simulink model "PubIfDecisionLM_MDL"  (R2020b)
settings: configuration reference "DspaceConfig" (kept outside this file)
PostLoadFcn:
  | if any(exist('dsrtsu_mdlpostloadfcn', 'file') ~= 0), dsrtsu_mdlpostloadfcn('Execute', bdroot); end
InitFcn:
  | , if any(exist('dsmpb_private', 'file') ~= 0), dsmpb_private('dsmpb_mdlclblib', 'Init', bdroot); end,
undefined symbols (not defined in the file or in its folder): OFM_OBJ_FUSIONTYPE_E, OFM_OBJ_MOVINGSTATE_E, OFM_OBJ_ORIENTATION_E, OFM_OBJ_TYPE_E, P_LM_Cyc, P_LM_EMLHistKapRcdBufSize, P_LM_EMLHistTrajBaseDis, P_LM_EMLHistTrajPNum, P_LM_EMLKapCorrMaxThre, P_LM_EMLMinKapThre, P_LM_EMLPathDisDiffThre, P_LM_EMLQuaFiltPar, P_LM_EMLTurnActKapThre, P_LM_EMLValidQuaThre, P_LM_FntPath1Disgap, P_LM_FntPath1MinDis, P_LM_FntPath1Timegap, P_LM_FntPath2Disgap, P_LM_FntPath2MinDis, P_LM_FntPath2Timegap, P_LM_FntPath3Disgap, P_LM_FntPath3MinDis, P_LM_FntPath3Timegap, P_LM_FusBLParFiltP, P_LM_FusEVDifC2Thre, P_LM_FusEVOPath1AllVSLDisThre, P_LM_FusEVOPath1AllVSLLostNumThre, P_LM_FusEVOPath1AllVSLQuaThre, P_LM_FusEVOPath1OTLFacNLC, P_LM_FusOTLQuaThre, P_LM_FusOTLSW, P_LM_FusParC0Index, P_LM_FusParC1Index, P_LM_FusParC2Index, P_LM_FusParC3Index, P_LM_FusVSLQuaThre, P_LM_FusVSLSW, P_LM_FusVSLValidSteerWheerAngThre, P_LM_FusVSLValidVxvThre, P_LM_LaneWidth, P_LM_OTLBufTPInfoEvaFactor, P_LM_OTLObjNum, P_LM_OTLObjSelectAgeThre, P_LM_OTLObjSelectDxAssessVx, P_LM_OTLObjSelectDxThre, P_LM_OTLObjSelectVxThre, P_LM_OTLObjSelectVyAssessDx, P_LM_OTLObjSelectVyThre, P_LM_OTLTrajPntBaseDis, P_LM_OTLTrajStdThre, P_LM_VSLAvailLineNum, P_LM_VSLBLSDiffThre, P_LM_VSLBLSDisRatio, P_LM_VSLFusBLParFiltP_C1, P_LM_VSLFusBLParFiltP_C2, P_LM_VSLFusBLParFiltP_C3, P_LM_VSLFusBLParFiltP_Quality, P_LM_VSLHistTrajBaseDis, P_LM_VSLHistTrajPNum, P_LM_VSLLCC0diff ... (+18)
libraries: simulink x145, LM_LIB x43
(part 10 of 24)

== system PubIfDecisionLM_MDL/Subsystem2/LM_SigPrePro1/Subsystem1/Subsystem/Subsystem2 ==
  RFM_LINE : Inport
  Bus Creator : BusCreator  Inputs=13
  Bus Selector : BusSelector  OutputSignals=dC0V
  Bus Selector1 : BusSelector  OutputSignals=bIsLineExist,dC1V,dC2V,dC3V,dLaneWidth,eLineType,dDisStart,dDisFront,dQuality,eColour,eFuType,nTrackAge
  Constant4 : Constant  Value=P_LM_VSLMinLINEL2  OutDataTypeStr=single
  Constant5 : Constant  Value=P_LM_VSLMaxLINEL2  OutDataTypeStr=single
  Constant8 : Constant  Value=0  OutDataTypeStr=single
  Logical Operator : Logic  AllPortsSameDT=off  OutDataTypeStr=boolean
  Relational Operator : RelationalOperator  OutDataTypeStr=boolean  RndMeth=Simplest
  Relational Operator1 : RelationalOperator  Operator=<=  OutDataTypeStr=boolean  RndMeth=Simplest
  Switch : Switch  Criteria=u2 > Threshold
  RFM_LINE_L2 : Outport
  wires:
  Relational Operator1/1 -> Logical Operator/2
  Bus Selector1/6 -> Bus Creator/7  "<eLineType>"
  Bus Selector1/8 -> Bus Creator/9  "<dDisFront>"
  Bus Selector1/5 -> Bus Creator/6  "<dLaneWidth>"
  Bus Selector1/9 -> Bus Creator/10  "<dQuality>"
  RFM_LINE/1 -> Bus Selector/1, Bus Selector1/1
  Logical Operator/1 -> Switch/2
  Bus Selector1/1 -> Bus Creator/1  "<bIsLineExist>"
  Bus Selector1/10 -> Bus Creator/11  "<eColour>"
  Bus Selector1/7 -> Bus Creator/8  "<dDisStart>"
  Bus Selector/1 -> Relational Operator1/1, Relational Operator/1, Switch/1  "<dC0V>"
  Switch/1 -> [dC0V]  "dC0V"
  Bus Selector1/3 -> Bus Creator/4  "<dC2V>"
  Bus Selector1/4 -> Bus Creator/5  "<dC3V>"
  Constant5/1 -> Relational Operator1/2
  Relational Operator/1 -> Logical Operator/1
  Constant8/1 -> Switch/3
  Bus Selector1/2 -> Bus Creator/3  "<dC1V>"
  [dC0V] -> Bus Creator/2  "dC0V"
  Constant4/1 -> Relational Operator/2
  Bus Creator/1 -> RFM_LINE_L2/1
  Bus Selector1/11 -> Bus Creator/12  "<eFuType>"
  Bus Selector1/12 -> Bus Creator/13  "<nTrackAge>"

== system PubIfDecisionLM_MDL/Subsystem2/LM_SigPrePro1/Subsystem1/Subsystem/Subsystem3 ==
  RFM_LINE : Inport
  Bus Creator : BusCreator  Inputs=13
  Bus Selector : BusSelector  OutputSignals=dC0V
  Bus Selector1 : BusSelector  OutputSignals=bIsLineExist,dC1V,dC2V,dC3V,dLaneWidth,eLineType,dDisStart,dDisFront,dQuality,eColour,eFuType,nTrackAge
  Constant6 : Constant  Value=P_LM_VSLMinLINER2  OutDataTypeStr=single
  Constant7 : Constant  Value=P_LM_VSLMaxLINER2  OutDataTypeStr=single
  Constant8 : Constant  Value=0  OutDataTypeStr=single
  Logical Operator : Logic  AllPortsSameDT=off  OutDataTypeStr=boolean
  Relational Operator : RelationalOperator  OutDataTypeStr=boolean  RndMeth=Simplest
  Relational Operator1 : RelationalOperator  Operator=<=  OutDataTypeStr=boolean  RndMeth=Simplest
  Switch : Switch  Criteria=u2 > Threshold
  RFM_LINE_R2 : Outport
  wires:
  Bus Creator/1 -> RFM_LINE_R2/1
  Constant6/1 -> Relational Operator/2
  [dC0V] -> Bus Creator/2  "dC0V"
  Bus Selector1/2 -> Bus Creator/3  "<dC1V>"
  Constant8/1 -> Switch/3
  Relational Operator/1 -> Logical Operator/1
  Constant7/1 -> Relational Operator1/2
  Bus Selector1/4 -> Bus Creator/5  "<dC3V>"
  Bus Selector1/3 -> Bus Creator/4  "<dC2V>"
  Switch/1 -> [dC0V]  "dC0V"
  Bus Selector/1 -> Switch/1, Relational Operator/1, Relational Operator1/1  "<dC0V>"
  Bus Selector1/7 -> Bus Creator/8  "<dDisStart>"
  Bus Selector1/10 -> Bus Creator/11  "<eColour>"
  Bus Selector1/1 -> Bus Creator/1  "<bIsLineExist>"
  Logical Operator/1 -> Switch/2
  RFM_LINE/1 -> Bus Selector1/1, Bus Selector/1
  Bus Selector1/9 -> Bus Creator/10  "<dQuality>"
  Bus Selector1/5 -> Bus Creator/6  "<dLaneWidth>"
  Bus Selector1/8 -> Bus Creator/9  "<dDisFront>"
  Bus Selector1/6 -> Bus Creator/7  "<eLineType>"
  Relational Operator1/1 -> Logical Operator/2
  Bus Selector1/11 -> Bus Creator/12  "<eFuType>"
  Bus Selector1/12 -> Bus Creator/13  "<nTrackAge>"

== system PubIfDecisionLM_MDL/Subsystem2/LM_VSL/LM_VSLFntPath/LM_VSL_LineInfoEvalutaion/LM_VSL_BaseLinePCalc3 ==
  LM_ComLineLostNum : Inport
  LM_VSLLineQualityVect : Inport  Port=2
  LM_VSLLineC1Vect : Inport  Port=3
  LM_VSLLineC2Vect : Inport  Port=4
  LM_VSLLineC3Vect : Inport  Port=5
  LM_VSLLineMaxQualityIndex : Inport  Port=6
  LM_VSLLineMinQualityIndex : Inport  Port=7
  Diffnum : Inport  Port=8
  LM_VSLMinQualityLineValid : Inport  Port=9
  LM_VSLDiffValid : Inport  Port=10
  LM_VSLBLFntDis : Inport  Port=11
  LM_VSLLineDisFntVect : Inport  Port=12
  Subsystem : Subsystem
  Subsystem1 : Subsystem
  LM_VSLBaseC1 : Outport
  LM_VSLBaseC2 : Outport  Port=2
  LM_VSLBaseC3 : Outport  Port=3
  LM_VSLBaseQuality : Outport  Port=4
  wires:
  LM_VSLBLFntDis/1 -> Subsystem/12(LM_VSLBLFntDis)
  LM_VSLLineDisFntVect/1 -> Subsystem/11(LM_VSLLineDisFntVect)
  Subsystem1/4(LM_VSLBaseQualityFilt) -> LM_VSLBaseQuality/1  "LM_VSLBaseQualityFilt"
  Subsystem1/3(LM_VSLBaseC3Filt) -> LM_VSLBaseC3/1  "LM_VSLBaseC3Filt"
  Subsystem1/2(LM_VSLBaseC2Filt) -> LM_VSLBaseC2/1  "LM_VSLBaseC2Filt"
  Subsystem1/1(LM_VSLBaseC1Filt) -> LM_VSLBaseC1/1  "LM_VSLBaseC1Filt"
  Subsystem/4(LM_VSLBaseQuality) -> Subsystem1/4(LM_VSLBaseQuality)  "LM_VSLBaseQuality"
  Subsystem/3(LM_VSLBaseC3) -> Subsystem1/3(LM_VSLBaseC3)  "LM_VSLBaseC3"
  Subsystem/2(LM_VSLBaseC2) -> Subsystem1/2(LM_VSLBaseC2)  "LM_VSLBaseC2"
  Subsystem/1(LM_VSLBaseC1) -> Subsystem1/1(LM_VSLBaseC1)  "LM_VSLBaseC1"
  LM_VSLLineMaxQualityIndex/1 -> Subsystem/1(LM_VSLLineMaxQualityIndex)
  LM_VSLLineQualityVect/1 -> Subsystem/7(LM_VSLLineQualityVect)
  LM_VSLMinQualityLineValid/1 -> Subsystem/10(LM_VSLMinQualityLineValid)
  LM_VSLLineC1Vect/1 -> Subsystem/4(LM_VSLLineC1Vect)
  LM_VSLLineC2Vect/1 -> Subsystem/5(LM_VSLLineC2Vect)
  LM_VSLLineC3Vect/1 -> Subsystem/6(LM_VSLLineC3Vect)
  LM_ComLineLostNum/1 -> Subsystem/3(LM_ComLineLostNum)
  LM_VSLLineMinQualityIndex/1 -> Subsystem/2(LM_VSLLineMinQualityIndex)
  LM_VSLDiffValid/1 -> Subsystem/9(LM_VSLDiffValid)
  Diffnum/1 -> Subsystem/8(Diffnum)

== system PubIfDecisionLM_MDL/Subsystem2/LM_VSL/LM_VSLFntPath/LM_VSL_LineInfoEvalutaion/LM_VSL_LineInfoEvalutaion ==
  LM_ComLineLostNum : Inport
  LM_VSLLineQualityVect : Inport  Port=2
  LM_VSLLineC1Vect : Inport  Port=3
  LM_VSLLineC2Vect : Inport  Port=4
  LM_VSLLineC3Vect : Inport  Port=5
  LM_VSLLineC0Vect : Inport  Port=6
  LM_ComAllLineLost_flg : Inport  Port=7
  LM_VSLLineExistVect : Inport  Port=8
  LM_VSLLineDisFntVect : Inport  Port=9
  LM_VSL_LineDiffEvalutaion : Subsystem
  LM_VSL_LineDisEvaluation : Subsystem
  LM_VSL_LineQualityEvalutaion : Subsystem
  LM_VSLLineMaxQualityIndex : Outport
  LM_VSLLineMinQualityIndex : Outport  Port=2
  Diffnum : Outport  Port=3
  LM_VSLMinQualityLineValid : Outport  Port=4
  LM_VSLDiffValid : Outport  Port=5
  LM_VSLBLFntDis : Outport  Port=6
  LM_VSLLineMaxDis : Outport  Port=7
  wires:
  LM_VSL_LineDiffEvalutaion/3(LM_VSLBLFntDis) -> LM_VSLBLFntDis/1
  LM_VSL_LineDisEvaluation/1(LM_VSLLineMaxDis) -> [LM_VSLLineMaxDis], LM_VSLLineMaxDis/1
  LM_ComAllLineLost_flg/1 -> LM_VSL_LineDisEvaluation/1(LM_ComAllLineLost_flg), LM_VSL_LineQualityEvalutaion/1(LM_ComAllLineLost_flg)
  LM_VSLLineQualityVect/1 -> LM_VSL_LineQualityEvalutaion/3(LM_VSLLineQualityVect), LM_VSL_LineDiffEvalutaion/2(LM_VSLLineQualityVect)
  LM_VSL_LineQualityEvalutaion/2(LM_VSLLineMaxQualityIndex) -> [LM_VSLLineMaxQualityIndex], LM_VSLLineMaxQualityIndex/1
  LM_VSL_LineQualityEvalutaion/1(LM_VSLLineMinQualityIndex) -> LM_VSLLineMinQualityIndex/1
  LM_ComLineLostNum/1 -> LM_VSL_LineDiffEvalutaion/4(LM_ComLineLostNum)
  LM_VSLLineC1Vect/1 -> LM_VSL_LineDiffEvalutaion/6(LM_VSLLineC1Vect)
  LM_VSLLineC2Vect/1 -> LM_VSL_LineDiffEvalutaion/7(LM_VSLLineC2Vect)
  LM_VSLLineC3Vect/1 -> LM_VSL_LineDiffEvalutaion/8(LM_VSLLineC3Vect)
  LM_VSL_LineDiffEvalutaion/1("Diffnum ") -> Diffnum/1
  LM_VSL_LineDiffEvalutaion/2(LM_VSLDiffValid) -> LM_VSLDiffValid/1
  LM_VSLLineC0Vect/1 -> LM_VSL_LineDiffEvalutaion/5(LM_VSLLineC0Vect)
  LM_VSLLineExistVect/1 -> LM_VSL_LineDisEvaluation/2(LM_VSLLineExistVect), LM_VSL_LineDiffEvalutaion/1(LM_VSLLineExistVect), LM_VSL_LineQualityEvalutaion/2(LM_VSLLineExistVect)
  LM_VSLLineDisFntVect/1 -> LM_VSL_LineDisEvaluation/3(LM_VSLLineDisFntVect), LM_VSL_LineDiffEvalutaion/3(LM_VSLLineDisFntVect)
  LM_VSL_LineQualityEvalutaion/3(LM_VSLLineMaxQuality) -> [LM_VSLLineMaxQuality]
  LM_VSL_LineDisEvaluation/2(LM_VSLLineMaxDisIndex) -> [LM_VSLLineMaxDisIndex]
  [LM_VSLLineMaxDisIndex] -> LM_VSL_LineDiffEvalutaion/11(LM_VSLLineMaxDisIndex)
  [LM_VSLLineMaxDis] -> LM_VSL_LineDiffEvalutaion/10(LM_VSLLineMaxDis)
  [LM_VSLLineMaxQualityIndex] -> LM_VSL_LineDiffEvalutaion/12(LM_VSLLineMaxQualityIndex)
  [LM_VSLLineMaxQuality] -> LM_VSL_LineDiffEvalutaion/9(LM_VSLLineMaxQuality)
  LM_VSL_LineQualityEvalutaion/4(LM_VSLMinQualityLineValid) -> LM_VSLMinQualityLineValid/1

== system PubIfDecisionLM_MDL/Subsystem2/LM_VSL/LM_VSLFntPath/LM_VSL_LineQualityCalc/LM_VSL_FntPath1QualityCalc ==
  LM_VSLBaseDisAdju : Inport
  LM_FntPath1Dis : Inport  Port=2
  LM_VSLBaseQuality : Inport  Port=3
  Divide : Product  Inputs=*/
  Product : Product
  Saturation : Saturate  UpperLimit=1  LowerLimit=0
  Saturation1 : Saturate  UpperLimit=1  LowerLimit=0
  Saturation2 : Saturate  UpperLimit=70  LowerLimit=5
  LM_VSLFntPath1Quality : Outport
  wires:
  Saturation2/1 -> Divide/1
  LM_FntPath1Dis/1 -> Divide/2
  Product/1 -> Saturation/1
  LM_VSLBaseDisAdju/1 -> Saturation2/1
  Saturation/1 -> LM_VSLFntPath1Quality/1  "LM_VSLFntPath1Quality"
  Saturation1/1 -> Product/1
  LM_VSLBaseQuality/1 -> Product/2
  Divide/1 -> Saturation1/1

== system PubIfDecisionLM_MDL/Subsystem2/LM_VSL/LM_VSLFntPath/LM_VSL_LineQualityCalc/LM_VSL_FntPath2QualityCalc ==
  LM_FntPath1Dis : Inport
  LM_VSLBaseQuality : Inport  Port=2
  LM_VSLBaseDis : Inport  Port=3
  LM_FntPath2Dis : Inport  Port=4
  Chart : Stateflow chart  TreatAsAtomicUnit=on
  Constant2 : Constant  Value=P_LM_VSLPath1DisDiffThre
  Signal Conversion : SignalConversion  OverrideOpt=off
  LM_VSLFntPath2Quality : Outport
  wires:
  Signal Conversion/1 -> LM_VSLFntPath2Quality/1  "LM_VSLFntPath2Quality"
  LM_FntPath2Dis/1 -> Chart/2(LM_FntPath2Dis)
  LM_VSLBaseQuality/1 -> Chart/4(LM_VSLBaseQuality)
  LM_VSLBaseDis/1 -> Chart/1(LM_VSLBaseDis)
  LM_FntPath1Dis/1 -> Chart/3(LM_FntPath1Dis)
  Constant2/1 -> Chart/5(P_LM_PathDisDiffThre)
  Chart/1(pathquality) -> Signal Conversion/1

== system PubIfDecisionLM_MDL/Subsystem2/LM_VSL/LM_VSLFntPath/LM_VSL_LineQualityCalc/LM_VSL_FntPath2QualityCalc1 ==
  note: 为了防止第二段轨迹短暂丢失，该处设计逻辑为当上一周期存在第二段，但本周期车道线长度不足输出第二段，会对第二段延迟半秒时间
  note: 为了避免车道线最大长度跳变导致一会儿有第2段一会儿又没第2段，可能会导致目标跳变，该处加入有效性校验，即第2段延后0.5s放出
  LM_FntPath1Dis : Inport
  LM_VSLBaseQuality : Inport  Port=2
  LM_VSLBaseDis : Inport  Port=3
  LM_FntPath2Dis : Inport  Port=4
  Add : Sum
  Add1 : Sum
  Compare To Constant : simulink/Logic and Bit Operations/Compare To Constant  relop===  const=1  OutDataTypeStr=boolean
  Compare To Zero : simulink/Logic and Bit Operations/Compare To Zero  relop=~=  OutDataTypeStr=boolean
  Compare To Zero1 : simulink/Logic and Bit Operations/Compare To Zero  relop=~=  OutDataTypeStr=boolean
  Compare To Zero2 : simulink/Logic and Bit Operations/Compare To Zero  relop===  OutDataTypeStr=boolean
  Constant : Constant  Value=0  OutDataTypeStr=single
  Constant1 : Constant  OutDataTypeStr=uint8
  Constant2 : Constant  Value=-5
  Constant3 : Constant  Value=15  OutDataTypeStr=uint8
  Constant4 : Constant  Value=0  OutDataTypeStr=uint8
  Constant5 : Constant  Commented=on  Value=P_LM_EMLPathDisDiffThre
  Constant6 : Constant  OutDataTypeStr=uint8
  Constant7 : Constant  Value=25  OutDataTypeStr=uint8
  Constant8 : Constant  OutDataTypeStr=uint8
  Constant9 : Constant  Value=25  OutDataTypeStr=uint8
  Divide : Product  Inputs=*/
  Logical Operator : Logic  AllPortsSameDT=off  OutDataTypeStr=boolean
  Logical Operator1 : Logic  AllPortsSameDT=off  OutDataTypeStr=boolean
  Logical Operator2 : Logic  Operator=OR  AllPortsSameDT=off  OutDataTypeStr=boolean
  Logical Operator3 : Logic  AllPortsSameDT=off  OutDataTypeStr=boolean
  Product : Product
  Relational Operator : RelationalOperator  OutDataTypeStr=boolean  RndMeth=Nearest
  Relational Operator1 : RelationalOperator  OutDataTypeStr=boolean  RndMeth=Nearest
  Relational Operator2 : RelationalOperator  Operator=<  OutDataTypeStr=boolean  RndMeth=Nearest
  Saturation : Saturate  UpperLimit=1  LowerLimit=0
  Saturation1 : Saturate  UpperLimit=1  LowerLimit=0
  Saturation2 : Saturate  UpperLimit=255  LowerLimit=0
  Saturation3 : Saturate  UpperLimit=253  LowerLimit=0
  Scope6 : Scope
  Subtract : Sum  Inputs=+-
  Switch{3..7} (5 alike) : Switch  Criteria=u2 ~= 0
  Unit Delay : UnitDelay  SampleTime=-1  HasFrameUpgradeWarning=on
  Unit Delay1 : UnitDelay  SampleTime=-1  HasFrameUpgradeWarning=on
  Unit Delay2 : UnitDelay  SampleTime=-1  HasFrameUpgradeWarning=on
  LM_VSLFntPath2Quality : Outport
  wires:
  Product/1 -> Saturation/1
  Switch5/1 -> Saturation2/1, Unit Delay/1
  Unit Delay2/1 -> Add1/2
  LM_VSLBaseDis/1 -> Compare To Zero/1, Subtract/1, Divide/1
  Switch6/1 -> Compare To Constant/1
  Divide/1 -> Saturation1/1
  Switch3/1 -> LM_VSLFntPath2Quality/1  "LM_VSLFntPath2Quality"
  LM_VSLBaseQuality/1 -> Product/2
  Subtract/1 -> Relational Operator/1
  Constant3/1 -> Relational Operator1/2
  Constant/1 -> Switch3/3
  LM_FntPath1Dis/1 -> Subtract/2
  Switch4/1 -> Switch5/1
  Constant2/1 -> Relational Operator/2
  Saturation2/1 -> Relational Operator1/1
  Constant4/1 -> Switch5/3
  Add/1 -> Switch4/1
  Compare To Zero/1 -> Logical Operator/2
  Constant1/1 -> Add/1
  Saturation1/1 -> Product/1
  Logical Operator2/1 -> Switch3/2
  LM_FntPath2Dis/1 -> Divide/2
  Compare To Constant/1 -> Switch7/2
  Logical Operator3/1 -> Switch6/2
  Constant7/1 -> Switch6/3
  Unit Delay/1 -> Add/2, Switch4/3
  Constant6/1 -> Switch6/1
  Switch7/1 -> Saturation3/1
  Constant9/1 -> Relational Operator2/2
  Compare To Zero1/1 -> Logical Operator3/1
  Saturation3/1 -> Relational Operator2/1, Unit Delay2/1, Scope6/1
  Relational Operator2/1 -> Logical Operator2/1
  Logical Operator1/1 -> Unit Delay1/1, Compare To Zero2/1, Logical Operator2/2
  Compare To Zero2/1 -> Logical Operator3/2
  Constant8/1 -> Switch7/1, Add1/1
  Add1/1 -> Switch7/3
  Relational Operator/1 -> Logical Operator/1
  Unit Delay1/1 -> Compare To Zero1/1
  Saturation/1 -> Switch3/1  "LM_VSL_FntPath2_Quality"
  Relational Operator1/1 -> Logical Operator1/2
  Logical Operator/1 -> Switch4/2, Logical Operator1/1, Switch5/2

== system PubIfDecisionLM_MDL/Subsystem2/LM_VSL/LM_VSLFntPath/LM_VSL_LineQualityCalc/LM_VSL_FntPath3QualityCalc ==
  note: 为了避免车道线最大长度跳变导致一会儿有第三段一会儿又没第三段，可能会导致目标跳变，该处加入有效性校验，即第三段延后0.5s放出
  LM_FntPath2Dis : Inport
  LM_VSLBaseQuality : Inport  Port=2
  LM_VSLBaseDis : Inport  Port=3
  LM_FntPath3Dis : Inport  Port=4
  Chart : Stateflow chart  TreatAsAtomicUnit=on
  Constant1 : Constant  Value=P_LM_VSLPath2DisDiffThre
  Signal Conversion : SignalConversion  OverrideOpt=off
  LM_VSLFntPath3Quality : Outport
  wires:
  Signal Conversion/1 -> LM_VSLFntPath3Quality/1  "LM_VSLFntPath3Quality"
  Constant1/1 -> Chart/5(P_LM_PathDisDiffThre)
  LM_FntPath3Dis/1 -> Chart/3(LM_FntPath3Dis)
  LM_VSLBaseQuality/1 -> Chart/4(LM_VSLBaseQuality)
  LM_FntPath2Dis/1 -> Chart/2(LM_FntPath2Dis)
  LM_VSLBaseDis/1 -> Chart/1(LM_VSLBaseDis)
  Chart/1(pathquality) -> Signal Conversion/1

== system PubIfDecisionLM_MDL/Subsystem2/LM_VSL/LM_VSLFntPath/LM_VSL_LineQualityCalc/LM_VSL_FntPath3QualityCalc1 ==
  note: 为了防止第二段轨迹短暂丢失，该处设计逻辑为当上一周期存在第二段，但本周期车道线长度不足输出第二段，会对第二段延迟半秒时间
  note: 为了避免车道线最大长度跳变导致一会儿有第三段一会儿又没第三段，可能会导致目标跳变，该处加入有效性校验，即第三段延后0.5s放出
  LM_FntPath2Dis : Inport
  LM_VSLBaseQuality : Inport  Port=2
  LM_VSLBaseDis : Inport  Port=3
  LM_FntPath3Dis : Inport  Port=4
  Add : Sum
  Add1 : Sum
  Chart : Stateflow chart  TreatAsAtomicUnit=on
  Compare To Constant : simulink/Logic and Bit Operations/Compare To Constant  relop===  const=1  OutDataTypeStr=boolean
  Compare To Zero : simulink/Logic and Bit Operations/Compare To Zero  relop=~=  OutDataTypeStr=boolean
  Compare To Zero1 : simulink/Logic and Bit Operations/Compare To Zero  relop=~=  OutDataTypeStr=boolean
  Compare To Zero2 : simulink/Logic and Bit Operations/Compare To Zero  relop===  OutDataTypeStr=boolean
  Constant : Constant  Value=0  OutDataTypeStr=single
  Constant1 : Constant  Value=-P_LM_EMLPathDisDiffThre
  Constant2 : Constant  OutDataTypeStr=uint8
  Constant3 : Constant  Value=10  OutDataTypeStr=uint8
  Constant4 : Constant  Value=0  OutDataTypeStr=uint8
  Constant6 : Constant  OutDataTypeStr=uint8
  Constant7 : Constant  Value=20  OutDataTypeStr=uint8
  Constant8 : Constant  OutDataTypeStr=uint8
  Constant9 : Constant  Value=20  OutDataTypeStr=uint8
  Divide : Product  Inputs=*/
  Logical Operator : Logic  AllPortsSameDT=off  OutDataTypeStr=boolean
  Logical Operator1 : Logic  AllPortsSameDT=off  OutDataTypeStr=boolean
  Logical Operator2 : Logic  Operator=OR  AllPortsSameDT=off  OutDataTypeStr=boolean
  Logical Operator3 : Logic  AllPortsSameDT=off  OutDataTypeStr=boolean
  Product : Product
  Relational Operator : RelationalOperator  OutDataTypeStr=boolean  RndMeth=Nearest
  Relational Operator1 : RelationalOperator  OutDataTypeStr=boolean  RndMeth=Nearest
  Relational Operator2 : RelationalOperator  Operator=<  OutDataTypeStr=boolean  RndMeth=Nearest
  Saturation : Saturate  UpperLimit=1  LowerLimit=0
  Saturation1 : Saturate  UpperLimit=1  LowerLimit=0
  Saturation2 : Saturate  UpperLimit=255  LowerLimit=0
  Saturation3 : Saturate  UpperLimit=253  LowerLimit=0
  Scope5 : Scope
  Subtract : Sum  Inputs=+-
  Switch{3..7} (5 alike) : Switch  Criteria=u2 ~= 0
  Unit Delay : UnitDelay  SampleTime=-1  HasFrameUpgradeWarning=on
  Unit Delay1 : UnitDelay  SampleTime=-1  HasFrameUpgradeWarning=on
  Unit Delay2 : UnitDelay  SampleTime=-1  HasFrameUpgradeWarning=on
  LM_VSLFntPath3Quality : Outport
  wires:
  LM_VSLBaseQuality/1 -> Product/2
  Saturation1/1 -> Product/1
  Product/1 -> Saturation/1
  Relational Operator/1 -> Logical Operator/1
  Subtract/1 -> Relational Operator/1
  Add/1 -> Switch4/1
  LM_VSLBaseDis/1 -> Compare To Zero/1, Divide/1, Subtract/1
  Constant1/1 -> Relational Operator/2
  Switch3/1 -> LM_VSLFntPath3Quality/1  "LM_VSLFntPath3Quality"
  Logical Operator2/1 -> Switch3/2
  LM_FntPath2Dis/1 -> Subtract/2, Scope5/1
  Saturation/1 -> Switch3/1  "LM_EML_FntPath3_Quality"
  Constant/1 -> Switch3/3
  Constant3/1 -> Relational Operator1/2
  LM_FntPath3Dis/1 -> Divide/2
  Compare To Zero2/1 -> Logical Operator3/2
  Compare To Constant/1 -> Switch7/2
  Switch5/1 -> Saturation2/1, Unit Delay/1
  Constant4/1 -> Switch5/3
  Switch6/1 -> Compare To Constant/1
  Compare To Zero/1 -> Logical Operator/2
  Divide/1 -> Saturation1/1
  Unit Delay/1 -> Add/2, Switch4/3
  Switch4/1 -> Switch5/1
  Saturation2/1 -> Relational Operator1/1
  Saturation3/1 -> Relational Operator2/1, Unit Delay2/1
  Constant8/1 -> Add1/1, Switch7/1
  Compare To Zero1/1 -> Logical Operator3/1
  Unit Delay2/1 -> Add1/2
  Unit Delay1/1 -> Compare To Zero1/1
  Relational Operator1/1 -> Logical Operator1/2
  Constant2/1 -> Add/1
  Relational Operator2/1 -> Logical Operator2/1
  Add1/1 -> Switch7/3
  Switch7/1 -> Saturation3/1
  Logical Operator/1 -> Logical Operator1/1, Switch5/2, Switch4/2
  Constant6/1 -> Switch6/1
  Constant7/1 -> Switch6/3
  Logical Operator1/1 -> Logical Operator2/2, Compare To Zero2/1, Unit Delay1/1
  Logical Operator3/1 -> Switch6/2
  Constant9/1 -> Relational Operator2/2

== system PubIfDecisionLM_MDL/Subsystem2/LM_VSL/LM_VSLRearPath/LM_VSLC0Calc/LM_RFMLineInfo ==
  LM_RFML2dC0V : Inport
  LM_RFML1dC0V : Inport  Port=2
  LM_RFMR1dC0V : Inport  Port=3
  LM_RFMR2dC0V : Inport  Port=4
  LM_RFML2IsLineExist : Inport  Port=5
  LM_RFML1IsLineExist : Inport  Port=6
  LM_RFMR1IsLineExist : Inport  Port=7
  LM_RFMR2IsLineExist : Inport  Port=8
  LM_RFML2dQuality : Inport  Port=9
  LM_RFML1dQuality : Inport  Port=10
  LM_RFMR1dQuality : Inport  Port=11
  LM_RFMR2dQuality : Inport  Port=12
  Mux : Mux
  Mux1 : Mux
  Mux2 : Mux
  RFM_VSLLineC0Vect : Outport
  RFM_VSLLineblsLineExistVect : Outport  Port=2
  RFM_VSLLineblsQualityVect : Outport  Port=3
  wires:
  Mux/1 -> RFM_VSLLineC0Vect/1
  LM_RFML2dC0V/1 -> Mux/1
  LM_RFML1dC0V/1 -> Mux/2
  LM_RFMR2dC0V/1 -> Mux/4
  LM_RFMR1dC0V/1 -> Mux/3
  Mux1/1 -> RFM_VSLLineblsLineExistVect/1
  Mux2/1 -> RFM_VSLLineblsQualityVect/1
  LM_RFMR1IsLineExist/1 -> Mux1/3
  LM_RFMR2IsLineExist/1 -> Mux1/4
  LM_RFML1IsLineExist/1 -> Mux1/2
  LM_RFML2IsLineExist/1 -> Mux1/1
  LM_RFML2dQuality/1 -> Mux2/1
  LM_RFML1dQuality/1 -> Mux2/2
  LM_RFMR2dQuality/1 -> Mux2/4
  LM_RFMR1dQuality/1 -> Mux2/3

== system PubIfDecisionLM_MDL/Subsystem2/LM_VSL/LM_VSLRearPath/LM_VSLHistLineInfoCoordinateConvert/If Action Subsystem ==
  LM_EMLOffsetX : Inport
  LM_EMLOffsetY : Inport  Port=2
  LM_EMLOffsetAng : Inport  Port=3
  LM_VSLLRC0HistInfoXK1 : Inport  Port=4
  LM_VSLLRC0HistInfoYK1 : Inport  Port=5
  LM_VSLRLC0HistInfoXK1 : Inport  Port=6
  LM_VSLRLC0HistInfoYK1 : Inport  Port=7
  Action Port : ActionPort  ActionPortLabel=if(u1 == 0)
  For Each Subsystem : Subsystem  TreatAsAtomicUnit=on
  LM_VSLLRC0HistInfoXK1Adju : Outport
  LM_VSLLRC0HistInfoYK1Adju : Outport  Port=2
  LM_VSLRLC0HistInfoXK1Adju : Outport  Port=3
  LM_VSLRLC0HistInfoYK1Adju : Outport  Port=4
  wires:
  LM_EMLOffsetX/1 -> For Each Subsystem/1(LM_EMLOffsetX)
  LM_EMLOffsetY/1 -> For Each Subsystem/2(LM_EMLOffsetY)
  LM_EMLOffsetAng/1 -> For Each Subsystem/3(LM_EMLOffsetAng)
  LM_VSLLRC0HistInfoYK1/1 -> For Each Subsystem/5(LM_VSLLRC0HistInfoYK1)
  LM_VSLLRC0HistInfoXK1/1 -> For Each Subsystem/4(LM_VSLLRC0HistInfoXK1)
  LM_VSLRLC0HistInfoXK1/1 -> For Each Subsystem/6(LM_VSLRLC0HistInfoXK1)
  LM_VSLRLC0HistInfoYK1/1 -> For Each Subsystem/7(LM_VSLRLC0HistInfoYK1)
  For Each Subsystem/2(LM_VSLLRC0HistInfoYK1Adju) -> LM_VSLLRC0HistInfoYK1Adju/1
  For Each Subsystem/1(LM_VSLLRC0HistInfoXK1Adju) -> LM_VSLLRC0HistInfoXK1Adju/1
  For Each Subsystem/4(LM_VSLRLC0HistInfoYK1Adju) -> LM_VSLRLC0HistInfoYK1Adju/1
  For Each Subsystem/3(LM_VSLRLC0HistInfoXK1Adju) -> LM_VSLRLC0HistInfoXK1Adju/1

== system PubIfDecisionLM_MDL/Subsystem2/LM_VSL/LM_VSLRearPath/LM_VSLHistLineInfoCoordinateConvert/If Action Subsystem1 ==
  LM_VSLLRC0HistInfoXK1 : Inport
  LM_VSLLRC0HistInfoYK1 : Inport  Port=2
  LM_VSLRLC0HistInfoXK1 : Inport  Port=3
  LM_VSLRLC0HistInfoYK1 : Inport  Port=4
  Action Port : ActionPort  ActionPortLabel=else
  LM_VSLLRC0HistInfoXK1Adju : Outport
  LM_VSLLRC0HistInfoYK1Adju : Outport  Port=2
  LM_VSLRLC0HistInfoXK1Adju : Outport  Port=3
  LM_VSLRLC0HistInfoYK1Adju : Outport  Port=4
  wires:
  LM_VSLRLC0HistInfoYK1/1 -> LM_VSLRLC0HistInfoYK1Adju/1
  LM_VSLRLC0HistInfoXK1/1 -> LM_VSLRLC0HistInfoXK1Adju/1
  LM_VSLLRC0HistInfoYK1/1 -> LM_VSLLRC0HistInfoYK1Adju/1
  LM_VSLLRC0HistInfoXK1/1 -> LM_VSLLRC0HistInfoXK1Adju/1

== system PubIfDecisionLM_MDL/Subsystem2/DIR/DrivingIntentionRecognition1/DIR_LaneChangeProbCalc/DIR_LaneChangeLeftProbCalc/If Action Subsystem ==
  DIR_LeftTurnLampOnTime : Inport
  SteerWheelAngle : Inport  Port=2
  SteerWheelAngleSign : Inport  Port=3
  LeftTurnSWSts : Inport  Port=4
  LM_LRC0 : Inport  Port=5
  LM_RLC0 : Inport  Port=6
  LM_VSLFntPathBaseC1 : Inport  Port=7
  Action Port : ActionPort  ActionPortLabel=if(u1 ~= 0)
  DIR_LaneChgLeProbByC1 : Subsystem
  DIR_LaneChgLeProbByLaneInfo : Subsystem
  DIR_LaneChgLeProbByLeftTurnSWSts : Subsystem
  DIR_LaneChgLeProbCalc : Subsystem
  DIR_LaneChgLeProbCalcBySteer : Subsystem
  DIR_tLC2LeValid : Outport
  wires:
  DIR_LaneChgLeProbByLaneInfo/1(DIR_LC2LeProbByLaneBorder) -> DIR_LaneChgLeProbCalc/2(DIR_LC2LeProbByLaneBorder)
  LeftTurnSWSts/1 -> DIR_LaneChgLeProbByLeftTurnSWSts/1(LeftTurnSWSts)
  LM_RLC0/1 -> DIR_LaneChgLeProbByLaneInfo/2(LM_RLC0)
  DIR_LaneChgLeProbCalc/1(DIR_tLC2LeValid) -> DIR_tLC2LeValid/1
  SteerWheelAngleSign/1 -> DIR_LaneChgLeProbCalcBySteer/3(SteerWheelAngleSign)
  LM_LRC0/1 -> DIR_LaneChgLeProbByLaneInfo/1(LM_LRC0)
  DIR_LaneChgLeProbCalcBySteer/1(DIR_LC2LeProbBySteer) -> DIR_LaneChgLeProbCalc/1(DIR_LC2LeProbBySteer)
  DIR_LaneChgLeProbByLeftTurnSWSts/1(DIR_LC2LeProbByTurnLampSts) -> DIR_LaneChgLeProbCalc/3(DIR_LC2LeProbByTurnLampSts)
  DIR_LeftTurnLampOnTime/1 -> DIR_LaneChgLeProbCalcBySteer/1(DIR_LeftTurnLampOnTime)
  SteerWheelAngle/1 -> DIR_LaneChgLeProbCalcBySteer/2(SteerWheelAngle)  "SteerWheelAngle"
  LM_VSLFntPathBaseC1/1 -> DIR_LaneChgLeProbByC1/1(LM_VSLFntPathBaseC1)
  DIR_LaneChgLeProbByC1/1(DIR_LaneChgLeByLineC1Valid) -> DIR_LaneChgLeProbCalc/4(DIR_LaneChgLeByLineC1Valid)

== system PubIfDecisionLM_MDL/Subsystem2/DIR/DrivingIntentionRecognition1/DIR_LaneChangeProbCalc/DIR_LaneChangeLeftProbCalc/If Action Subsystem1 ==
  SteerWheelAngle : Inport
  SteerWheelAngleSign : Inport  Port=2
  LM_LRC0 : Inport  Port=3
  LM_RLC0 : Inport  Port=4
  LM_VSLFntPathBaseC1 : Inport  Port=5
  DIR_EgoVehOnLineValid : Inport  Port=6
  vxvRefMs : Inport  Port=7
  Action Port : ActionPort  ActionPortLabel=else
  DIR_LaneChgLeProbByLaneInfo : Subsystem
  DIR_LaneChgLeProbByLaneInfo1 : Subsystem
  DIR_LaneChgLeProbCalc : Subsystem
  DIR_LaneChgLeProbCalcBySteer : Subsystem
  DIR_tLC2LeValid : Outport
  wires:
  SteerWheelAngle/1 -> DIR_LaneChgLeProbCalcBySteer/1(SteerWheelAngle)  "SteerWheelAngle"
  DIR_LaneChgLeProbCalcBySteer/1(DIR_LaneChgLeBySteerValid) -> DIR_LaneChgLeProbCalc/1(DIR_LC2LeProbBySteer)
  DIR_LaneChgLeProbByLaneInfo/1(DIR_LaneChgLeByLaneBorderValid) -> DIR_LaneChgLeProbCalc/2(DIR_LC2LeProbByLaneBorder)
  DIR_LaneChgLeProbCalc/1(DIR_tLC2LeValid) -> DIR_tLC2LeValid/1
  LM_RLC0/1 -> DIR_LaneChgLeProbByLaneInfo/2(LM_RLC0)
  SteerWheelAngleSign/1 -> DIR_LaneChgLeProbCalcBySteer/2(SteerWheelAngleSign)
  LM_LRC0/1 -> DIR_LaneChgLeProbByLaneInfo/1(LM_LRC0)
  vxvRefMs/1 -> DIR_LaneChgLeProbCalcBySteer/4(vxvRefMs)
  DIR_EgoVehOnLineValid/1 -> DIR_LaneChgLeProbCalcBySteer/3(DIR_EgoVehOnLineValid)
  LM_VSLFntPathBaseC1/1 -> DIR_LaneChgLeProbByLaneInfo1/1(LM_VSLFntPathBaseC1)
  DIR_LaneChgLeProbByLaneInfo1/1(DIR_LaneChgLeByLineC1Valid) -> DIR_LaneChgLeProbCalc/3(DIR_LaneChgLeByLineC1Valid)

== system PubIfDecisionLM_MDL/Subsystem2/DIR/DrivingIntentionRecognition1/DIR_LaneChangeProbCalc/DIR_LaneChangeLeftProbCalc/Subsystem1 ==
  DIR_tLC2LeValid : Inport
  Add : Sum
  Constant : Constant  OutDataTypeStr=int8
  Constant1 : Constant  Value=-1  OutDataTypeStr=int8
  Constant2 : Constant  Value=10  OutDataTypeStr=int8
  Constant3 : Constant  Value=50  OutDataTypeStr=int8
  Product : Product
  Relational Operator : RelationalOperator  OutDataTypeStr=boolean  RndMeth=Simplest
  Saturation : Saturate  UpperLimit=100  LowerLimit=0
  Switch : Switch  Criteria=u2 ~= 0
  Unit Delay : UnitDelay  SampleTime=-1  HasFrameUpgradeWarning=on
  DIR_LC2LeValid : Outport
  wires:
  Relational Operator/1 -> DIR_LC2LeValid/1  "DIR_LC2LeValid"
  Constant3/1 -> Relational Operator/2
  Saturation/1 -> Relational Operator/1, Unit Delay/1
  Add/1 -> Saturation/1
  Unit Delay/1 -> Add/2
  Product/1 -> Add/1
  Constant2/1 -> Product/2
  Switch/1 -> Product/1
  Constant1/1 -> Switch/3
  Constant/1 -> Switch/1
  DIR_tLC2LeValid/1 -> Switch/2

== system PubIfDecisionLM_MDL/Subsystem2/DIR/DrivingIntentionRecognition1/DIR_LaneChangeProbCalc/DIR_LaneChangeRightProbCalc/If Action Subsystem ==
  RightTurnSWSts : Inport
  DIR_RightTurnLampOnTime : Inport  Port=2
  SteerWheelAngle : Inport  Port=3
  SteerWheelAngleSign : Inport  Port=4
  LM_LRC0 : Inport  Port=5
  LM_RLC0 : Inport  Port=6
  LM_VSLFntPathBaseC1 : Inport  Port=7
  Action Port : ActionPort  ActionPortLabel=if(u1 ~= 0)
  DIR_LaneChgLeProbByLaneInfo : Subsystem
  DIR_LaneChgLeProbByLaneInfo1 : Subsystem
  DIR_LaneChgLeProbByLeftTurnSWSts : Subsystem
  DIR_LaneChgLeProbCalc : Subsystem
  DIR_LaneChgLeProbCalcBySteer : Subsystem
  DIR_tLC2RigValid : Outport
  wires:
  SteerWheelAngle/1 -> DIR_LaneChgLeProbCalcBySteer/2(SteerWheelAngle)  "SteerWheelAngle"
  DIR_RightTurnLampOnTime/1 -> DIR_LaneChgLeProbCalcBySteer/1(DIR_RightTurnLampOnTime)
  DIR_LaneChgLeProbByLeftTurnSWSts/1(DIR_LC2RigProbByTurnLampSts) -> DIR_LaneChgLeProbCalc/3(DIR_LC2RigProbByTurnLampSts)
  DIR_LaneChgLeProbCalcBySteer/1(DIR_LC2LeProbBySteer) -> DIR_LaneChgLeProbCalc/1(DIR_LC2RigProbBySteer)
  LM_LRC0/1 -> DIR_LaneChgLeProbByLaneInfo/1(LM_LRC0)
  SteerWheelAngleSign/1 -> DIR_LaneChgLeProbCalcBySteer/3(SteerWheelAngleSign)
  DIR_LaneChgLeProbCalc/1(DIR_tLC2RigValid) -> DIR_tLC2RigValid/1
  LM_RLC0/1 -> DIR_LaneChgLeProbByLaneInfo/2(LM_RLC0)
  RightTurnSWSts/1 -> DIR_LaneChgLeProbByLeftTurnSWSts/1(RightTurnSWSts)
  DIR_LaneChgLeProbByLaneInfo/1(DIR_LC2LeProbByLaneBorder) -> DIR_LaneChgLeProbCalc/2(DIR_LC2RigProbByLaneBorder)
  LM_VSLFntPathBaseC1/1 -> DIR_LaneChgLeProbByLaneInfo1/1(LM_VSLFntPathBaseC1)
  DIR_LaneChgLeProbByLaneInfo1/1(DIR_LaneChgRigByLineC1Valid) -> DIR_LaneChgLeProbCalc/4(DIR_LaneChgRigByLineC1Valid)

== system PubIfDecisionLM_MDL/Subsystem2/DIR/DrivingIntentionRecognition1/DIR_LaneChangeProbCalc/DIR_LaneChangeRightProbCalc/If Action Subsystem1 ==
  SteerWheelAngle : Inport
  SteerWheelAngleSign : Inport  Port=2
  LM_LRC0 : Inport  Port=3
  LM_RLC0 : Inport  Port=4
  LM_VSLFntPathBaseC1 : Inport  Port=5
  DIR_EgoVehOnLineValid : Inport  Port=6
  vxvRefMs : Inport  Port=7
  Action Port : ActionPort  ActionPortLabel=else
  DIR_LaneChgLeProbByLaneInfo : Subsystem
  DIR_LaneChgLeProbByLaneInfo1 : Subsystem
  DIR_LaneChgLeProbCalc : Subsystem
  DIR_LaneChgLeProbCalcBySteer : Subsystem
  DIR_tLC2RigValid : Outport
  wires:
  DIR_LaneChgLeProbByLaneInfo1/1(DIR_LaneChgRigByLineC1Valid) -> DIR_LaneChgLeProbCalc/3(DIR_LaneChgRigByLineC1Valid)
  LM_VSLFntPathBaseC1/1 -> DIR_LaneChgLeProbByLaneInfo1/1(LM_VSLFntPathBaseC1)
  DIR_EgoVehOnLineValid/1 -> DIR_LaneChgLeProbCalcBySteer/3(DIR_EgoVehOnLineValid)
  vxvRefMs/1 -> DIR_LaneChgLeProbCalcBySteer/4(vxvRefMs)
  LM_LRC0/1 -> DIR_LaneChgLeProbByLaneInfo/1(LM_LRC0)
  SteerWheelAngleSign/1 -> DIR_LaneChgLeProbCalcBySteer/2(SteerWheelAngleSign)
  LM_RLC0/1 -> DIR_LaneChgLeProbByLaneInfo/2(LM_RLC0)
  DIR_LaneChgLeProbCalc/1(DIR_tLC2RigValid) -> DIR_tLC2RigValid/1
  DIR_LaneChgLeProbByLaneInfo/1(DIR_LaneChgRigByLaneBorderValid) -> DIR_LaneChgLeProbCalc/2(DIR_LC2RjgProbByLaneBorder)
  DIR_LaneChgLeProbCalcBySteer/1(DIR_LaneChgRigBySteerValid) -> DIR_LaneChgLeProbCalc/1(DIR_LC2RigProbBySteer)
  SteerWheelAngle/1 -> DIR_LaneChgLeProbCalcBySteer/1(SteerWheelAngle)  "SteerWheelAngle"

== system PubIfDecisionLM_MDL/Subsystem2/DIR/DrivingIntentionRecognition1/DIR_TurnDirProbCalc/DIR_TurnLeftProbCalc/DIR_TurnLeftProbByTurnLampOnTime ==
  DIR_LeftTurnLampOnTime : Inport
  1-D Lookup Table : Lookup_n-D  NumberOfTableDimensions=1  BreakpointsForDimension1=[0,1,2,3]  Table=[0,0.33,0.67,1]  InternalRulePriority=Speed  RndMeth=Simplest  InputSameDT=on
  Constant : Constant  Value=3  OutDataTypeStr=single
  Constant1 : Constant  OutDataTypeStr=single
  Constant2 : Constant  Value=0  OutDataTypeStr=single
  Constant3 : Constant  Value=0  OutDataTypeStr=single
  Logical Operator : Logic  AllPortsSameDT=off  OutDataTypeStr=boolean
  Relational Operator : RelationalOperator  OutDataTypeStr=boolean  RndMeth=Simplest
  Relational Operator1 : RelationalOperator  OutDataTypeStr=boolean  RndMeth=Simplest
  Relational Operator2 : RelationalOperator  Operator=<  OutDataTypeStr=boolean  RndMeth=Simplest
  Switch : Switch  Criteria=u2 ~= 0
  Switch1 : Switch  Criteria=u2 ~= 0
  DIR_TurnLeftProbBytTurnLamp : Outport
  wires:
  Switch/1 -> DIR_TurnLeftProbBytTurnLamp/1  "LM_DIRTurnLeftProbBytTurnLamp"
  Switch1/1 -> Switch/3
  Constant3/1 -> Switch1/3
  1-D Lookup Table/1 -> Switch1/1
  Logical Operator/1 -> Switch1/2
  Relational Operator1/1 -> Logical Operator/2
  Relational Operator2/1 -> Logical Operator/1
  Constant2/1 -> Relational Operator1/2
  Constant1/1 -> Switch/1
  Relational Operator/1 -> Switch/2
  Constant/1 -> Relational Operator2/2, Relational Operator/2
  DIR_LeftTurnLampOnTime/1 -> Relational Operator/1, 1-D Lookup Table/1, Relational Operator1/1, Relational Operator2/1

== system PubIfDecisionLM_MDL/Subsystem2/DIR/DrivingIntentionRecognition1/DIR_TurnDirProbCalc/DIR_TurnLeftProbCalc/DIR_TurnLeftProbCalc ==
  DIR_TurnLeftProbBytTurnLamp : Inport
  DIR_TurnLeftProbByTurnLampSts : Inport  Port=2
  DIR_TurnLeftProbByVehSpd : Inport  Port=3
  DIR_TurnLeftProbByPsiDtopt : Inport  Port=4
  DIR_TurnLeftProbByKapTraj : Inport  Port=5
  DIR_TurnLeftProbBySteerWheelAng : Inport  Port=6
  Add : Sum
  Add1 : Sum
  Constant : Constant  Value=0.1  OutDataTypeStr=single
  Constant1 : Constant  Value=0.75  OutDataTypeStr=single
  Constant10 : Constant  OutDataTypeStr=boolean
  Constant2 : Constant  Value=0.25  OutDataTypeStr=single
  Constant3 : Constant  Value=0.85  OutDataTypeStr=single
  Constant4 : Constant  OutDataTypeStr=int8
  Constant5 : Constant  Value=-1  OutDataTypeStr=int8
  Constant6 : Constant  Value=10  OutDataTypeStr=int8
  Constant7 : Constant  Value=50  OutDataTypeStr=int8
  Constant8 : Constant  Value=0.58  OutDataTypeStr=single
  Constant9 : Constant  Value=0  OutDataTypeStr=boolean
  Logical Operator : Logic  Operator=OR  AllPortsSameDT=off  OutDataTypeStr=boolean
  MinMax : MinMax  Inputs=6
  Product : Product
  Product1 : Product
  Relational Operator : RelationalOperator  Operator=>  OutDataTypeStr=boolean  RndMeth=Simplest
  Relational Operator1 : RelationalOperator  OutDataTypeStr=boolean  RndMeth=Simplest
  Relational Operator2 : RelationalOperator  OutDataTypeStr=boolean  RndMeth=Simplest
  Relational Operator3 : RelationalOperator  Operator=>  OutDataTypeStr=boolean  RndMeth=Simplest
  Saturation : Saturate  UpperLimit=100  LowerLimit=0
  Switch : Switch  Criteria=u2 ~= 0
  Switch1 : Switch  Criteria=u2 ~= 0
  Switch2 : Switch  Criteria=u2 ~= 0
  Unit Delay2 : UnitDelay  SampleTime=-1  HasFrameUpgradeWarning=on
  DIR_TurnLeftValid : Outport
  wires:
  Add/1 -> Switch/1
  Constant2/1 -> Product/2
  Product/1 -> Add/2
  Constant1/1 -> Add/1
  Switch/1 -> Relational Operator3/1  "LM_DIRTurnLeftProb"
  Constant/1 -> Relational Operator/2
  Relational Operator/1 -> Switch/2
  MinMax/1 -> Relational Operator/1, Product/1, Switch/3
  DIR_TurnLeftProbBySteerWheelAng/1 -> MinMax/6
  DIR_TurnLeftProbByKapTraj/1 -> Relational Operator1/1, MinMax/5
  DIR_TurnLeftProbByPsiDtopt/1 -> MinMax/4
  DIR_TurnLeftProbByVehSpd/1 -> MinMax/3
  DIR_TurnLeftProbByTurnLampSts/1 -> MinMax/2
  DIR_TurnLeftProbBytTurnLamp/1 -> MinMax/1
  Constant3/1 -> Relational Operator1/2
  Constant7/1 -> Relational Operator2/2
  Unit Delay2/1 -> Add1/2
  Constant5/1 -> Switch1/3
  Constant6/1 -> Product1/2
  Switch1/1 -> Product1/1
  Relational Operator1/1 -> Switch1/2
  Add1/1 -> Saturation/1
  Constant4/1 -> Switch1/1
  Product1/1 -> Add1/1
  Saturation/1 -> Unit Delay2/1, Relational Operator2/1
  Constant8/1 -> Relational Operator3/2
  Relational Operator3/1 -> Logical Operator/1
  Relational Operator2/1 -> Switch2/3
  Logical Operator/1 -> DIR_TurnLeftValid/1  "LM_DIRTurnLeftValid"
  Constant9/1 -> Switch2/1
  Constant10/1 -> Switch2/2
  Switch2/1 -> Logical Operator/2

== system PubIfDecisionLM_MDL/Subsystem2/DIR/DrivingIntentionRecognition1/DIR_TurnDirProbCalc/DIR_TurnLeftProbCalc/DIR_TurnLeftProbCalcByCurveKap ==
  kapTraj : Inport
  1-D Lookup Table : Lookup_n-D  NumberOfTableDimensions=1  BreakpointsForDimension1=[0.01,0.014,0.018,0.022,0.026]  Table=[0,0.25,0.5,0.75,1]  InternalRulePriority=Speed  RndMeth=Simplest  InputSameDT=on
  Constant : Constant  Value=0.026  OutDataTypeStr=single
  Constant1 : Constant  OutDataTypeStr=single
  Constant2 : Constant  Value=0.01  OutDataTypeStr=single
  Constant3 : Constant  Value=0  OutDataTypeStr=single
  Logical Operator : Logic  AllPortsSameDT=off  OutDataTypeStr=boolean
  Relational Operator : RelationalOperator  OutDataTypeStr=boolean  RndMeth=Simplest
  Relational Operator1 : RelationalOperator  Operator=<  OutDataTypeStr=boolean  RndMeth=Simplest
  Relational Operator2 : RelationalOperator  OutDataTypeStr=boolean  RndMeth=Simplest
  Switch : Switch  Criteria=u2 ~= 0
  Switch1 : Switch  Criteria=u2 ~= 0
  DIR_TurnLeftProbByKapTraj : Outport
  wires:
  1-D Lookup Table/1 -> Switch1/1
  Switch/1 -> DIR_TurnLeftProbByKapTraj/1  "LM_DIRTurnLeftProbByKapTraj"
  Relational Operator1/1 -> Logical Operator/1
  kapTraj/1 -> Relational Operator/1, Relational Operator1/1, Relational Operator2/1, 1-D Lookup Table/1
  Switch1/1 -> Switch/3
  Relational Operator/1 -> Switch/2
  Relational Operator2/1 -> Logical Operator/2
  Constant3/1 -> Switch1/3
  Constant/1 -> Relational Operator/2, Relational Operator1/2
  Constant1/1 -> Switch/1
  Logical Operator/1 -> Switch1/2
  Constant2/1 -> Relational Operator2/2

== system PubIfDecisionLM_MDL/Subsystem2/DIR/DrivingIntentionRecognition1/DIR_TurnDirProbCalc/DIR_TurnLeftProbCalc/DIR_TurnLeftProbCalcByPsiDtOpt ==
  PsiDtOpt : Inport
  1-D Lookup Table : Lookup_n-D  NumberOfTableDimensions=1  BreakpointsForDimension1=[0.11,0.15,0.19,0.23]  Table=[0,0.33,0.67,1]  InternalRulePriority=Speed  RndMeth=Simplest  InputSameDT=on
  Constant : Constant  Value=0.23  OutDataTypeStr=single
  Constant1 : Constant  OutDataTypeStr=single
  Constant2 : Constant  Value=0.11  OutDataTypeStr=single
  Constant3 : Constant  Value=0  OutDataTypeStr=single
  Logical Operator : Logic  AllPortsSameDT=off  OutDataTypeStr=boolean
  Relational Operator : RelationalOperator  OutDataTypeStr=boolean  RndMeth=Simplest
  Relational Operator1 : RelationalOperator  Operator=<  OutDataTypeStr=boolean  RndMeth=Simplest
  Relational Operator2 : RelationalOperator  OutDataTypeStr=boolean  RndMeth=Simplest
  Switch : Switch  Criteria=u2 ~= 0
  Switch1 : Switch  Criteria=u2 ~= 0
  DIR_TurnLeftProbByPsiDtopt : Outport
  wires:
  1-D Lookup Table/1 -> Switch1/1
  Switch/1 -> DIR_TurnLeftProbByPsiDtopt/1  "LM_DIRTurnLeftProbByPsiDtopt"
  Switch1/1 -> Switch/3
  Constant3/1 -> Switch1/3
  Logical Operator/1 -> Switch1/2
  Relational Operator2/1 -> Logical Operator/2
  Relational Operator1/1 -> Logical Operator/1
  Constant2/1 -> Relational Operator2/2
  Constant1/1 -> Switch/1
  Relational Operator/1 -> Switch/2
  Constant/1 -> Relational Operator/2, Relational Operator1/2
  PsiDtOpt/1 -> Relational Operator/1, Relational Operator1/1, Relational Operator2/1, 1-D Lookup Table/1

== system PubIfDecisionLM_MDL/Subsystem2/DIR/DrivingIntentionRecognition1/DIR_TurnDirProbCalc/DIR_TurnLeftProbCalc/DIR_TurnLeftProbCalcBySteerWheelAng ==
  SteerWheelAngle : Inport
  SteerWheelAngleSign : Inport  Port=2
  1-D Lookup Table : Lookup_n-D  NumberOfTableDimensions=1  BreakpointsForDimension1=[85,90,95,100]  Table=[0,0.33,0.67,1]  InternalRulePriority=Speed  RndMeth=Simplest  InputSameDT=on
  Constant : Constant  Value=100  OutDataTypeStr=single
  Constant1 : Constant  OutDataTypeStr=single
  Constant2 : Constant  Value=85  OutDataTypeStr=single
  Constant3 : Constant  Value=0  OutDataTypeStr=single
  Constant4 : Constant  Value=0  OutDataTypeStr=uint8
  Logical Operator : Logic  Inputs=3  AllPortsSameDT=off  OutDataTypeStr=boolean
  Logical Operator1 : Logic  AllPortsSameDT=off  OutDataTypeStr=boolean
  Relational Operator : RelationalOperator  OutDataTypeStr=boolean  RndMeth=Simplest
  Relational Operator1 : RelationalOperator  Operator=<  OutDataTypeStr=boolean  RndMeth=Simplest
  Relational Operator2 : RelationalOperator  OutDataTypeStr=boolean  RndMeth=Simplest
  Relational Operator3 : RelationalOperator  Operator===  OutDataTypeStr=boolean  RndMeth=Simplest
  Switch : Switch  Criteria=u2 ~= 0
  Switch1 : Switch  Criteria=u2 ~= 0
  DIR_TurnLeftProbBySteerWheelAng : Outport
  wires:
  [SteerLeftFlg] -> Logical Operator/3
  Logical Operator1/1 -> Switch/2
  Constant4/1 -> Relational Operator3/2
  SteerWheelAngleSign/1 -> Relational Operator3/1
  Relational Operator3/1 -> Logical Operator1/1, [SteerLeftFlg]
  1-D Lookup Table/1 -> Switch1/1
  Switch1/1 -> Switch/3
  Constant3/1 -> Switch1/3
  Constant1/1 -> Switch/1
  Logical Operator/1 -> Switch1/2
  Constant2/1 -> Relational Operator2/2
  Relational Operator/1 -> Logical Operator1/2
  Relational Operator2/1 -> Logical Operator/2
  Constant/1 -> Relational Operator1/2, Relational Operator/2
  Relational Operator1/1 -> Logical Operator/1
  Switch/1 -> DIR_TurnLeftProbBySteerWheelAng/1  "LM_DIRTurnLeftProbBySteerWheelAng"
  SteerWheelAngle/1 -> Relational Operator/1, Relational Operator1/1, Relational Operator2/1, 1-D Lookup Table/1

== system PubIfDecisionLM_MDL/Subsystem2/DIR/DrivingIntentionRecognition1/DIR_TurnDirProbCalc/DIR_TurnLeftProbCalc/DIR_TurnLeftProbCalcByTurnLampSts ==
  LeftTurnSWSts : Inport
  Constant : Constant  OutDataTypeStr=uint8
  Constant1 : Constant  OutDataTypeStr=single
  Constant2 : Constant  Value=0  OutDataTypeStr=single
  Relational Operator : RelationalOperator  Operator===  OutDataTypeStr=boolean  RndMeth=Simplest
  Switch : Switch  Criteria=u2 ~= 0
  DIR_TurnLeftProbByTurnLampSts : Outport
  wires:
  Switch/1 -> DIR_TurnLeftProbByTurnLampSts/1  "LM_DIRTurnLeftProbByTurnLampSts"
  Constant2/1 -> Switch/3
  Constant1/1 -> Switch/1
  Relational Operator/1 -> Switch/2
  Constant/1 -> Relational Operator/2
  LeftTurnSWSts/1 -> Relational Operator/1

== system PubIfDecisionLM_MDL/Subsystem2/DIR/DrivingIntentionRecognition1/DIR_TurnDirProbCalc/DIR_TurnLeftProbCalc/DIR_TurnLeftProbCalcByVehSpd ==
  vxvRefMs : Inport
  1-D Lookup Table : Lookup_n-D  NumberOfTableDimensions=1  BreakpointsForDimension1=[12,12.5,13,13.5,14]  Table=[1,0.75,0.5,0.25,0]  InternalRulePriority=Speed  RndMeth=Simplest  InputSameDT=on
  Constant : Constant  Value=12  OutDataTypeStr=single
  Constant1 : Constant  OutDataTypeStr=single
  Constant2 : Constant  Value=14  OutDataTypeStr=single
  Constant3 : Constant  Value=0  OutDataTypeStr=single
  Logical Operator : Logic  AllPortsSameDT=off  OutDataTypeStr=boolean
  Relational Operator : RelationalOperator  Operator=<=  OutDataTypeStr=boolean  RndMeth=Simplest
  Relational Operator1 : RelationalOperator  Operator=>  OutDataTypeStr=boolean  RndMeth=Simplest
  Relational Operator2 : RelationalOperator  Operator=<=  OutDataTypeStr=boolean  RndMeth=Simplest
  Signal Conversion : SignalConversion  OverrideOpt=off
  Switch : Switch  Criteria=u2 ~= 0
  Switch1 : Switch  Criteria=u2 ~= 0
  DIR_TurnLeftProbByVehSpd : Outport
  wires:
  Switch/1 -> Signal Conversion/1
  Constant3/1 -> Switch1/3
  1-D Lookup Table/1 -> Switch1/1
  Switch1/1 -> Switch/3
  Logical Operator/1 -> Switch1/2
  Relational Operator2/1 -> Logical Operator/2
  Relational Operator1/1 -> Logical Operator/1
  Constant2/1 -> Relational Operator2/2
  Relational Operator/1 -> Switch/2
  Constant1/1 -> Switch/1
  Constant/1 -> Relational Operator1/2, Relational Operator/2
  vxvRefMs/1 -> Relational Operator/1, 1-D Lookup Table/1, Relational Operator1/1, Relational Operator2/1
  Signal Conversion/1 -> DIR_TurnLeftProbByVehSpd/1  "LM_DIRTurnLeftProbByVehSpd"

== system PubIfDecisionLM_MDL/Subsystem2/DIR/DrivingIntentionRecognition1/DIR_TurnDirProbCalc/DIR_TurnRightProbCalc/DIR_TurnLeftProbCalc ==
  DIR_TurnRightProbBytTurnLamp : Inport
  DIR_TurnRightProbByTurnLampSts : Inport  Port=2
  DIR_TurnRightProbByVehSpd : Inport  Port=3
  DIR_TurnRightProbByPsiDtopt : Inport  Port=4
  DIR_TurnRightProbByKapTraj : Inport  Port=5
  DIR_TurnRightProbBySteerWheelAng : Inport  Port=6
  Add : Sum
  Add1 : Sum
  Constant : Constant  Value=0.1  OutDataTypeStr=single
  Constant1 : Constant  Value=0.5  OutDataTypeStr=single
  Constant10 : Constant  OutDataTypeStr=boolean
  Constant2 : Constant  Value=0.25  OutDataTypeStr=single
  Constant3 : Constant  Value=0.85  OutDataTypeStr=single
  Constant4 : Constant  OutDataTypeStr=int8
  Constant5 : Constant  Value=-1  OutDataTypeStr=int8
  Constant6 : Constant  Value=10  OutDataTypeStr=int8
  Constant7 : Constant  Value=50  OutDataTypeStr=int8
  Constant8 : Constant  Value=0.58  OutDataTypeStr=single
  Constant9 : Constant  Value=0  OutDataTypeStr=boolean
  Logical Operator : Logic  Operator=OR  AllPortsSameDT=off  OutDataTypeStr=boolean
  MinMax : MinMax  Inputs=6
  Product : Product
  Product1 : Product
  Relational Operator : RelationalOperator  Operator=>  OutDataTypeStr=boolean  RndMeth=Simplest
  Relational Operator1 : RelationalOperator  OutDataTypeStr=boolean  RndMeth=Simplest
  Relational Operator2 : RelationalOperator  OutDataTypeStr=boolean  RndMeth=Simplest
  Relational Operator3 : RelationalOperator  Operator=>  OutDataTypeStr=boolean  RndMeth=Simplest
  Saturation : Saturate  UpperLimit=100  LowerLimit=0
  Switch : Switch  Criteria=u2 ~= 0
  Switch1 : Switch  Criteria=u2 ~= 0
  Switch2 : Switch  Criteria=u2 ~= 0
  Unit Delay2 : UnitDelay  SampleTime=-1  HasFrameUpgradeWarning=on
  DIR_TurnRightValid : Outport
  wires:
  Add/1 -> Switch/1
  Constant2/1 -> Product/2
  Product/1 -> Add/2
  Constant1/1 -> Add/1
  Switch/1 -> Relational Operator3/1  "LM_DIRTurnRightProb"
  Constant/1 -> Relational Operator/2
  Relational Operator/1 -> Switch/2
  MinMax/1 -> Relational Operator/1, Product/1, Switch/3
  DIR_TurnRightProbBySteerWheelAng/1 -> MinMax/6
  DIR_TurnRightProbByPsiDtopt/1 -> MinMax/4
  DIR_TurnRightProbByVehSpd/1 -> MinMax/3
  DIR_TurnRightProbByTurnLampSts/1 -> MinMax/2
  DIR_TurnRightProbBytTurnLamp/1 -> MinMax/1
  Relational Operator1/1 -> Switch1/2
  DIR_TurnRightProbByKapTraj/1 -> Relational Operator1/1, MinMax/5
  Saturation/1 -> Unit Delay2/1, Relational Operator2/1
  Add1/1 -> Saturation/1
  Switch1/1 -> Product1/1
  Constant4/1 -> Switch1/1
  Product1/1 -> Add1/1
  Constant5/1 -> Switch1/3
  Unit Delay2/1 -> Add1/2
  Constant3/1 -> Relational Operator1/2
  Constant6/1 -> Product1/2
  Constant7/1 -> Relational Operator2/2
  Relational Operator3/1 -> Logical Operator/1
  Constant8/1 -> Relational Operator3/2
  Relational Operator2/1 -> Switch2/3
  Logical Operator/1 -> DIR_TurnRightValid/1  "LM_DIRTurnRightValid"
  Constant10/1 -> Switch2/2
  Constant9/1 -> Switch2/1
  Switch2/1 -> Logical Operator/2

== system PubIfDecisionLM_MDL/Subsystem2/DIR/DrivingIntentionRecognition1/DIR_TurnDirProbCalc/DIR_TurnRightProbCalc/DIR_TurnRightProbByTurnLampOnTime ==
  DIR_RightTurnLampOnTime : Inport
  1-D Lookup Table : Lookup_n-D  NumberOfTableDimensions=1  BreakpointsForDimension1=[0,1,2,3]  Table=[0,0.33,0.67,1]  InternalRulePriority=Speed  RndMeth=Simplest  InputSameDT=on
  Constant : Constant  Value=3  OutDataTypeStr=single
  Constant1 : Constant  OutDataTypeStr=single
  Constant2 : Constant  Value=0  OutDataTypeStr=single
  Constant3 : Constant  Value=0  OutDataTypeStr=single
  Logical Operator : Logic  AllPortsSameDT=off  OutDataTypeStr=boolean
  Relational Operator : RelationalOperator  OutDataTypeStr=boolean  RndMeth=Simplest
  Relational Operator1 : RelationalOperator  OutDataTypeStr=boolean  RndMeth=Simplest
  Relational Operator2 : RelationalOperator  Operator=<  OutDataTypeStr=boolean  RndMeth=Simplest
  Switch : Switch  Criteria=u2 ~= 0
  Switch1 : Switch  Criteria=u2 ~= 0
  DIR_TurnRightProbBytTurnLamp : Outport
  wires:
  Switch/1 -> DIR_TurnRightProbBytTurnLamp/1  "LM_DIRTurnRightProbBytTurnLamp"
  Switch1/1 -> Switch/3
  Constant3/1 -> Switch1/3
  1-D Lookup Table/1 -> Switch1/1
  Logical Operator/1 -> Switch1/2
  Relational Operator1/1 -> Logical Operator/2
  Relational Operator2/1 -> Logical Operator/1
  Constant2/1 -> Relational Operator1/2
  Constant1/1 -> Switch/1
  Relational Operator/1 -> Switch/2
  Constant/1 -> Relational Operator2/2, Relational Operator/2
  DIR_RightTurnLampOnTime/1 -> Relational Operator/1, 1-D Lookup Table/1, Relational Operator1/1, Relational Operator2/1
